simulink model "si5b_bouncing_ball_elastic"  (R2024a)
settings: Solver=VariableStepAuto  StartTime=0.0  StopTime=10  RelTol=1e-3
values from neighbouring files (symbols this model uses):
  c = -0.8    [si5_Ball_parameter.m]    (also in sim21_ODE.m = 1)
  g = 9.81    [Electromagnet_par.m]    (also in si5_Ball_parameter.m; sim21_eventsdemo_jumpingBall.m = -9.81)
  h = 10    [si5_Ball_parameter.m]
  k = 10    [si5_Ball_parameter.m]    (also in sim21_ODE.m = 3)
  m = 0.35    [Electromagnet_par.m]    (also in si5_Ball_parameter.m = 0.1; sim21_ODE.m = 3)
settings Model: Creator=ocean  LastModifiedBy=ocean

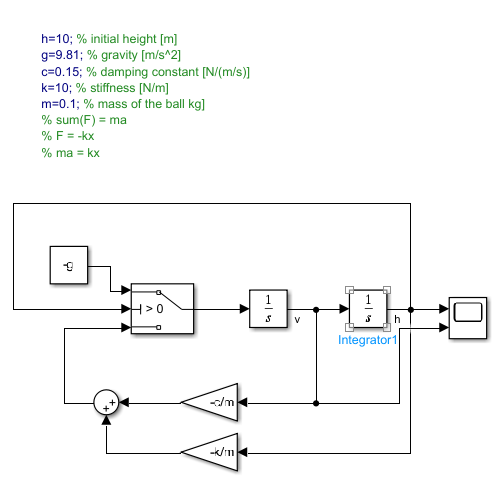
[thumbnail: Simulink's stored preview of the top-level diagram]
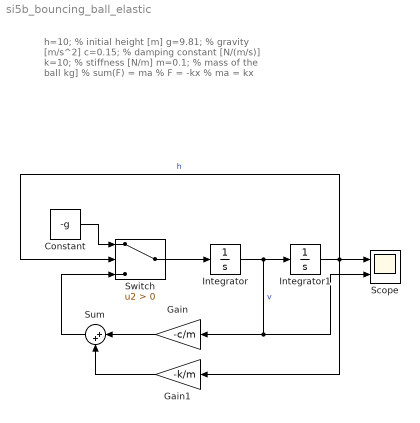
== system si5b_bouncing_ball_elastic ==
  note: h=10; % initial height [m]
      | g=9.81; % gravity [m/s^2]
      | c=0.15; % damping constant [N/(m/s)]
      | k=10; % stiffness [N/m]
      | m=0.1; % mass of the ball kg]
      | % sum(F) = ma
      | % F = -kx
      | % ma = kx
  Constant : Constant  Value=-g
  Gain : Gain  Gain=-c/m
  Gain1 : Gain  Gain=-k/m
  Integrator : Integrator
  Integrator1 : Integrator  InitialCondition=h
  Scope : Scope  NumInputPorts=2
  Sum : Sum  Inputs=|++
  Switch : Switch  Criteria=u2 > Threshold  SaturateOnIntegerOverflow=off  InputSameDT=off
  wires:
  Integrator/1 -> Scope/2, Gain/1, Integrator1/1  "v"
  Constant/1 -> Switch/1
  Integrator1/1 -> Switch/2, Gain1/1, Scope/1  "h"
  Switch/1 -> Integrator/1
  Gain1/1 -> Sum/2
  Gain/1 -> Sum/1
  Sum/1 -> Switch/3
